simulink model "LoadSaveScript_test"  (Simulink 6.2)
settings: Solver=FixedStepDiscrete  StartTime=0.0  StopTime=3  FixedStep=1  RelTol=1e-3
undefined symbols (not defined in the file or in its folder): param
libraries: LoadSaveScript_Lib x1
settings Model: LastModifiedBy=bsaunder
settings DebuggingCC: SolverPrmCheckMsg=warning

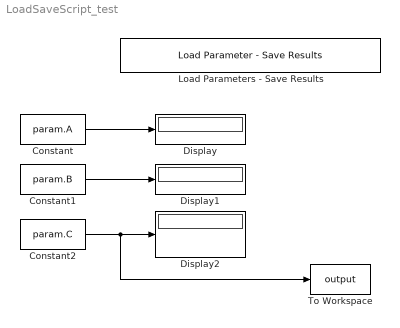
== system LoadSaveScript_test ==
  Constant : Constant  Value=param.A
  Constant1 : Constant  Value=param.B
  Constant2 : Constant  Value=param.C
  Display : Display
  Display1 : Display
  Display2 : Display
  Load Parameters - Save Results : LoadSaveScript_Lib/Load Parameter - Save Results  Priority=0
  To Workspace : ToWorkspace  VariableName=output  SampleTime=-1  SaveFormat=Array
  wires:
  Constant/1 -> Display/1
  Constant1/1 -> Display1/1
  Constant2/1 -> Display2/1, To Workspace/1
